simulink model "mvdc_path_matching"  (R2018b)
settings: configuration reference "Active" (kept outside this file)
undefined symbols (not defined in the file): P_VDC_ActivateHighPathDeviationDetection_b, P_VDC_CurvatureForesight_s, P_VDC_HeadingPathDeviationMax_rad, P_VDC_LateralPathDeviationMax_m, P_VDC_LocalFFCalculationActive_b, P_VDC_PathMatchForesight_m, P_VDC_PathMatchingTimeOut, P_VDC_PathMatchInterpPoints, P_VDC_PowertrainForesight_s, P_VDC_SmoothPathActive_b, P_VDC_SmoothPathWeights_DeltaCurvature, P_VDC_SmoothPathWeights_LatDeviation, tS, TUMPathMatchingState
libraries: simulink x5, rr_general x1
settings Model: DataDictionary=mvdc_path_matching.sldd  Creator=wischnewski  LastModifiedBy=ge34qer

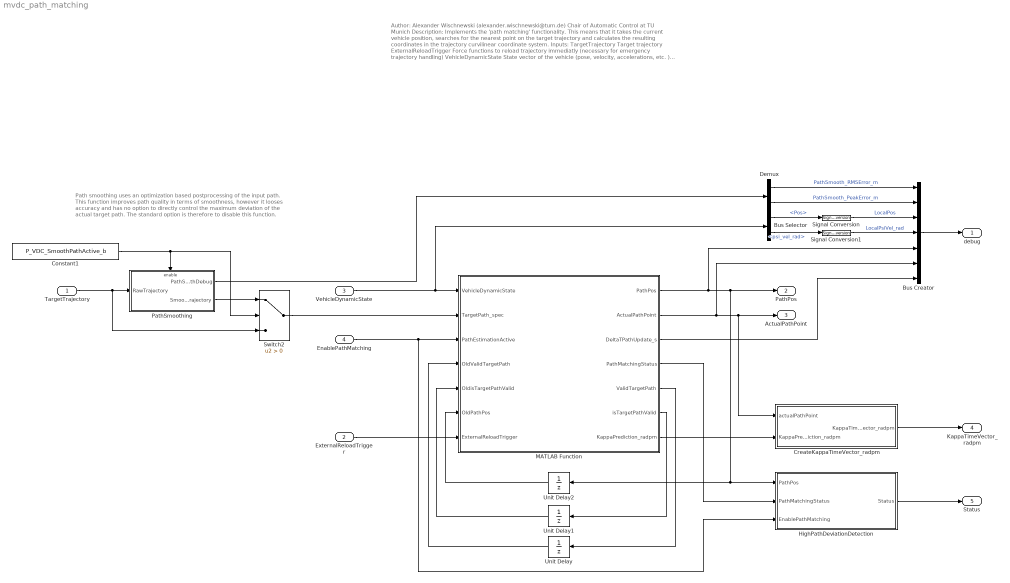
== system mvdc_path_matching ==
  note: Author: Alexander Wischnewski (alexander.wischnewski@tum.de)
      | Chair of Automatic Control at TU Munich
      |
      | Description: Implements the 'path matching' functionality. This means that it takes the current vehicle position, searches for
      | the nearest point on the target trajectory and calculates the resulting coordinates in the trajectory curvilinear
      | coordinate system.
      |
      | Inputs:
      | TargetTrajectory Target trajectory
      | ExternalReloadTrigger Force functions to reload trajectory immediatly (necessary for emergency trajectory handling)
      | VehicleDynamicState State vector of the vehicle (pose, velocity, accelerations, etc. )
      | EnablePathMatching Activates matching functionality
      |
      | Outputs:
      | debug debug bus
      | PathPos Vehicle position in path coordinates
      | ActualPathPoint Path on the target trajectory which is nearest to the vehicle
      | KappaTimeVector_radpm Vector which holds path curvature for a time window of +- 0.5sec
      | Status Function status used for state machine logic and diagnosis
  note: Path smoothing uses an optimization based postprocessing of the
      | input path. This function improves path quality in terms of smoothness,
      | however it looses accuracy and has no option to directly control the maximum deviation of the actual target path. The standard option is therefore to disable this function.
  TargetTrajectory : Inport  OutDataTypeStr=Bus: Trajectory  PortDimensions=1  Interpolate=off  BusOutputAsStruct=on
  ExternalReloadTrigger : Inport  Port=2  OutDataTypeStr=boolean  PortDimensions=1  BusOutputAsStruct=on
  VehicleDynamicState : Inport  Port=3  OutDataTypeStr=Bus: VehicleDynamicState  PortDimensions=1  BusOutputAsStruct=on
  EnablePathMatching : Inport  Port=4  OutDataTypeStr=boolean  PortDimensions=1  BusOutputAsStruct=on
  Bus Creator : BusCreator  Inputs=7  OutDataTypeStr=Bus: mvdc_path_matching_debug
  Bus Selector : BusSelector  OutputSignals=Pos,psi_vel_rad
  Constant1 : Constant  Value=P_VDC_SmoothPathActive_b
  CreateKappaTimeVector_radpm : Subsystem
  Demux : Demux  Outputs=2
  HighPathDeviationDetection : Subsystem
  MATLAB Function : MATLAB Function  TreatAsAtomicUnit=on
  PathSmoothing : Subsystem
  Signal Conversion : SignalConversion  OverrideOpt=off
  Signal Conversion1 : SignalConversion  OverrideOpt=off
  Switch2 : Switch  Criteria=u2 > Threshold
  Unit Delay : UnitDelay  SampleTime=-1
  Unit Delay1 : UnitDelay  SampleTime=-1
  Unit Delay2 : UnitDelay  SampleTime=-1
  debug : Outport  OutDataTypeStr=Bus: mvdc_path_matching_debug  PortDimensions=1  BusOutputAsStruct=on
  PathPos : Outport  Port=2  OutDataTypeStr=Bus: PathPos  PortDimensions=1  BusOutputAsStruct=on
  ActualPathPoint : Outport  Port=3  OutDataTypeStr=Bus: PathPoint  PortDimensions=1  BusOutputAsStruct=on
  KappaTimeVector_radpm : Outport  Port=4  PortDimensions=501
  Status : Outport  Port=5  OutDataTypeStr=Enum: TUMPathMatchingState  PortDimensions=1
  wires:
  MATLAB Function/1(PathPos) -> Unit Delay2/1, HighPathDeviationDetection/1(PathPos), PathPos/1, Bus Creator/5
  VehicleDynamicState/1 -> MATLAB Function/1(VehicleDynamicState), Bus Selector/1
  MATLAB Function/2(ActualPathPoint) -> CreateKappaTimeVector_radpm/1(actualPathPoint), ActualPathPoint/1, Bus Creator/6
  Bus Creator/1 -> debug/1
  MATLAB Function/3(DeltaTPathUpdate_s) -> Bus Creator/7
  HighPathDeviationDetection/1(Status) -> Status/1
  EnablePathMatching/1 -> HighPathDeviationDetection/3(EnablePathMatching), MATLAB Function/3(PathEstimationActive)
  Signal Conversion/1 -> Bus Creator/3  "LocalPos"
  MATLAB Function/5(ValidTargetPath) -> Unit Delay/1
  Unit Delay/1 -> MATLAB Function/4(OldValidTargetPath)
  MATLAB Function/6(isTargetPathValid) -> Unit Delay1/1
  Unit Delay1/1 -> MATLAB Function/5(OldisTargetPathValid)
  Unit Delay2/1 -> MATLAB Function/6(OldPathPos)
  Demux/1 -> Bus Creator/1  "PathSmooth_RMSError_m"
  Demux/2 -> Bus Creator/2  "PathSmooth_PeakError_m"
  Bus Selector/1 -> Signal Conversion/1  "<Pos>"
  Bus Selector/2 -> Signal Conversion1/1  "<psi_vel_rad>"
  Signal Conversion1/1 -> Bus Creator/4  "LocalPsiVel_rad"
  ExternalReloadTrigger/1 -> MATLAB Function/7(ExternalReloadTrigger)
  TargetTrajectory/1 -> Switch2/3, PathSmoothing/1(RawTrajectory)
  Constant1/1 -> Switch2/2, PathSmoothing/Enable
  PathSmoothing/2(SmoothTrajectory) -> Switch2/1
  Switch2/1 -> MATLAB Function/2(TargetPath_spec)
  PathSmoothing/1(PathSmoothDebug) -> Demux/1
  CreateKappaTimeVector_radpm/1(KappaTimeVector_radpm) -> KappaTimeVector_radpm/1
  MATLAB Function/7(KappaPrediction_radpm) -> CreateKappaTimeVector_radpm/2(KappaPrediction_radpm)
  MATLAB Function/4(PathMatchingStatus) -> HighPathDeviationDetection/2(PathMatchingStatus)

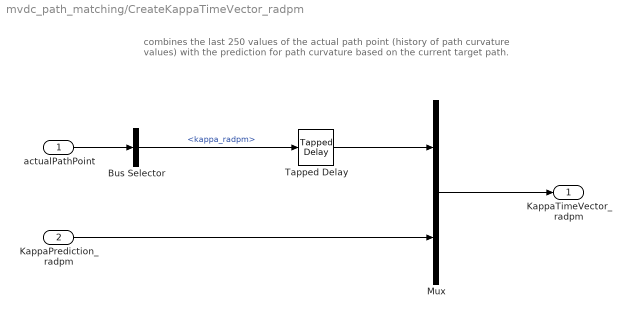
== system mvdc_path_matching/CreateKappaTimeVector_radpm ==
  note: combines the last 250 values of the actual path point (history of path curvature
      | values) with the prediction for path curvature based on the current target path.
  actualPathPoint : Inport
  KappaPrediction_radpm : Inport  Port=2
  Bus Selector : BusSelector  OutputSignals=kappa_radpm
  Mux : Mux  Inputs=2
  Tapped Delay : simulink/Discrete/Tapped Delay  vinit=0.0  samptime=-1  NumDelays=250  DelayOrder=Oldest  includeCurrent=off
  KappaTimeVector_radpm : Outport
  wires:
  Mux/1 -> KappaTimeVector_radpm/1
  KappaPrediction_radpm/1 -> Mux/2
  actualPathPoint/1 -> Bus Selector/1
  Bus Selector/1 -> Tapped Delay/1  "<kappa_radpm>"
  Tapped Delay/1 -> Mux/1

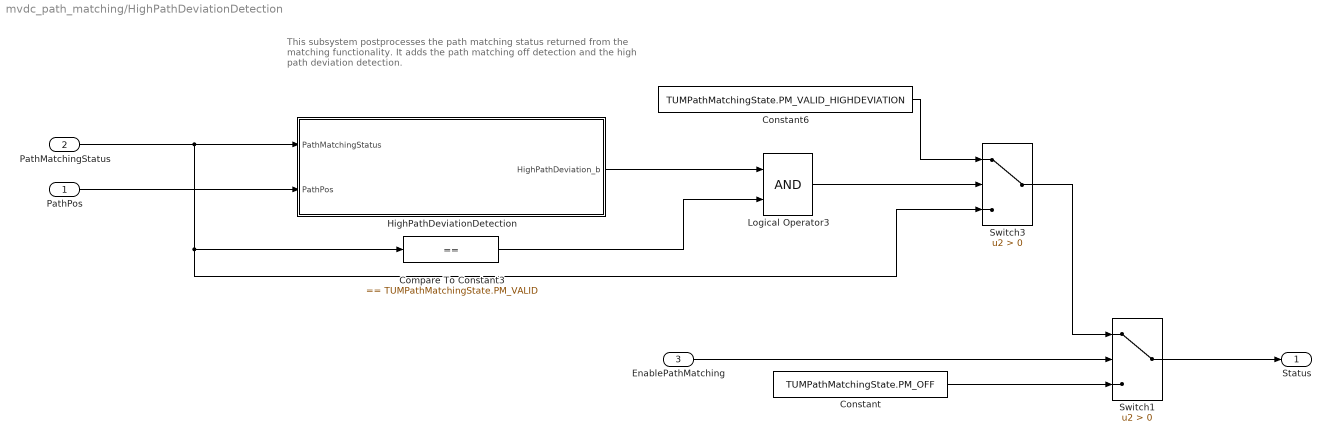
== system mvdc_path_matching/HighPathDeviationDetection ==
  note: This subsystem postprocesses the path matching status returned from the
      | matching functionality. It adds the path matching off detection and the
      | high path deviation detection.
  PathPos : Inport
  PathMatchingStatus : Inport  Port=2
  EnablePathMatching : Inport  Port=3
  Compare To Constant3 : simulink/Logic and Bit Operations/Compare To Constant  relop===  const=TUMPathMatchingState.PM_VALID  OutDataTypeStr=boolean
  Constant : Constant  Value=TUMPathMatchingState.PM_OFF
  Constant6 : Constant  Value=TUMPathMatchingState.PM_VALID_HIGHDEVIATION
  HighPathDeviationDetection : Subsystem
  Logical Operator3 : Logic  AllPortsSameDT=off  OutDataTypeStr=boolean
  Switch1 : Switch  Criteria=u2 > Threshold
  Switch3 : Switch  Criteria=u2 > Threshold
  Status : Outport  OutDataTypeStr=Enum: TUMPathMatchingState
  wires:
  EnablePathMatching/1 -> Switch1/2
  Constant/1 -> Switch1/3
  Switch1/1 -> Status/1
  Switch3/1 -> Switch1/1
  Logical Operator3/1 -> Switch3/2
  Compare To Constant3/1 -> Logical Operator3/2
  PathMatchingStatus/1 -> HighPathDeviationDetection/1(PathMatchingStatus), Switch3/3, Compare To Constant3/1
  PathPos/1 -> HighPathDeviationDetection/2(PathPos)
  HighPathDeviationDetection/1(HighPathDeviation_b) -> Logical Operator3/1
  Constant6/1 -> Switch3/1

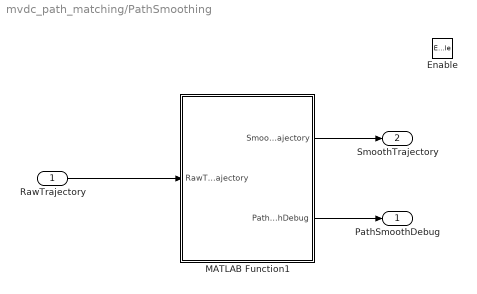
== system mvdc_path_matching/PathSmoothing ==
  RawTrajectory : Inport
  Enable : EnablePort
  MATLAB Function1 : MATLAB Function  TreatAsAtomicUnit=on
  PathSmoothDebug : Outport
  SmoothTrajectory : Outport  Port=2
  wires:
  MATLAB Function1/2(PathSmoothDebug) -> PathSmoothDebug/1
  MATLAB Function1/1(SmoothTrajectory) -> SmoothTrajectory/1
  RawTrajectory/1 -> MATLAB Function1/1(RawTrajectory)

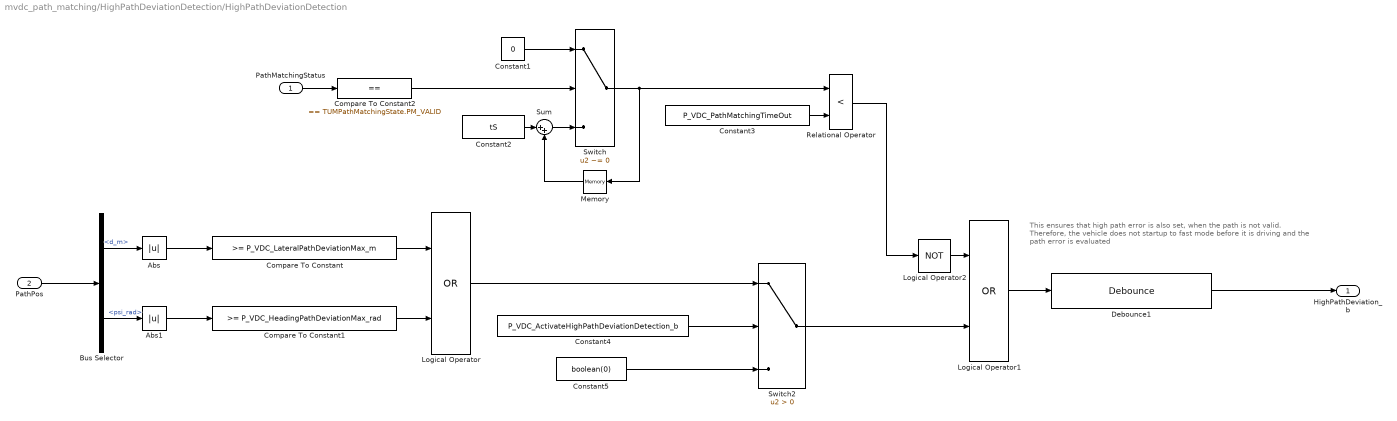
== system mvdc_path_matching/HighPathDeviationDetection/HighPathDeviationDetection ==
  note: This ensures that high path error is also set, when the path is not valid.
      | Therefore, the vehicle does not startup to fast mode before it is driving and
      | the path error is evaluated
  PathMatchingStatus : Inport
  PathPos : Inport  Port=2
  Abs : Abs
  Abs1 : Abs
  Bus Selector : BusSelector  OutputSignals=d_m,psi_rad
  Compare To Constant : simulink/Logic and Bit Operations/Compare To Constant  relop=>=  const=P_VDC_LateralPathDeviationMax_m  OutDataTypeStr=boolean
  Compare To Constant1 : simulink/Logic and Bit Operations/Compare To Constant  relop=>=  const=P_VDC_HeadingPathDeviationMax_rad  OutDataTypeStr=boolean
  Compare To Constant2 : simulink/Logic and Bit Operations/Compare To Constant  relop===  const=TUMPathMatchingState.PM_VALID  OutDataTypeStr=boolean
  Constant1 : Constant  Value=0
  Constant2 : Constant  Value=tS
  Constant3 : Constant  Value=P_VDC_PathMatchingTimeOut
  Constant4 : Constant  Value=P_VDC_ActivateHighPathDeviationDetection_b
  Constant5 : Constant  Value=boolean(0)
  Debounce1 : rr_general/Debounce  debounce_cycles=P_VDC_HighPathDeviationDebounce
  Logical Operator : Logic  Operator=OR  AllPortsSameDT=off  OutDataTypeStr=boolean
  Logical Operator1 : Logic  Operator=OR  AllPortsSameDT=off  OutDataTypeStr=boolean
  Logical Operator2 : Logic  Operator=NOT  AllPortsSameDT=off  OutDataTypeStr=boolean
  Memory : Memory  InitialCondition=P_VDC_PathMatchingTimeOut  InheritSampleTime=on
  Relational Operator : RelationalOperator  Operator=<  OutDataTypeStr=boolean  RndMeth=Nearest
  Sum : Sum  Inputs=|++
  Switch : Switch  Criteria=u2 ~= 0
  Switch2 : Switch  Criteria=u2 > Threshold
  HighPathDeviation_b : Outport
  wires:
  Switch/1 -> Memory/1, Relational Operator/1
  PathPos/1 -> Bus Selector/1
  Abs/1 -> Compare To Constant/1
  Logical Operator2/1 -> Logical Operator1/1
  Constant5/1 -> Switch2/3
  Logical Operator/1 -> Switch2/1
  Compare To Constant1/1 -> Logical Operator/2
  Constant4/1 -> Switch2/2
  Abs1/1 -> Compare To Constant1/1
  Compare To Constant/1 -> Logical Operator/1
  Sum/1 -> Switch/3
  Logical Operator1/1 -> Debounce1/1
  Relational Operator/1 -> Logical Operator2/1
  Bus Selector/1 -> Abs/1  "<d_m>"
  Switch2/1 -> Logical Operator1/2
  Debounce1/1 -> HighPathDeviation_b/1
  Bus Selector/2 -> Abs1/1  "<psi_rad>"
  Memory/1 -> Sum/2
  Constant3/1 -> Relational Operator/2
  Compare To Constant2/1 -> Switch/2
  Constant1/1 -> Switch/1
  Constant2/1 -> Sum/1
  PathMatchingStatus/1 -> Compare To Constant2/1

== matlab function mvdc_path_matching/PathSmoothing/MATLAB Function1 ==
  data: RawTrajectory input Bus: Trajectory; SmoothTrajectory output Bus: Trajectory; PathSmoothDebug output; P_VDC_SmoothPathWeights_LatDeviation parameter; P_VDC_SmoothPathWeights_DeltaCurvature parameter
function [SmoothTrajectory, PathSmoothDebug] = smoothRaceline(RawTrajectory, P_VDC_SmoothPathWeights_LatDeviation, P_VDC_SmoothPathWeights_DeltaCurvature)
  % wrapper function for smooth raceline
  [SmoothTrajectory, PathSmoothDebug] =...
  smoothRaceline(RawTrajectory, P_VDC_SmoothPathWeights_LatDeviation, P_VDC_SmoothPathWeights_DeltaCurvature);
end

== matlab function mvdc_path_matching/MATLAB Function ==
  data: VehicleDynamicState input Bus: VehicleDynamicState; TargetPath_spec input Bus: Trajectory; PathEstimationActive input boolean; OldValidTargetPath input Bus: Trajectory; OldisTargetPathValid input boolean; OldPathPos input Bus: PathPos; ExternalReloadTrigger input; PathPos output Bus: PathPos; tS parameter; ActualPathPoint output Bus: PathPoint; P_VDC_PathMatchInterpPoints parameter; P_VDC_PowertrainForesight_s parameter; P_VDC_CurvatureForesight_s parameter; P_VDC_LocalFFCalculationActive_b parameter; DeltaTPathUpdate_s output; P_VDC_PathMatchForesight_m parameter; PathMatchingStatus output Enum: TUMPathMatchingState; ValidTargetPath output Bus: Trajectory; isTargetPathValid output boolean size=1; KappaPrediction_radpm output size=251
function [PathPos, ActualPathPoint, DeltaTPathUpdate_s, PathMatchingStatus, ValidTargetPath, isTargetPathValid, KappaPrediction_radpm]  = mvdc_path_matching(VehicleDynamicState, TargetPath_spec, PathEstimationActive, OldValidTargetPath, OldisTargetPathValid, OldPathPos, ExternalReloadTrigger, tS, P_VDC_PathMatchInterpPoints, P_VDC_PowertrainForesight_s, P_VDC_CurvatureForesight_s, P_VDC_LocalFFCalculationActive_b, P_VDC_PathMatchForesight_m)
  [PathPos, ActualPathPoint, DeltaTPathUpdate_s, PathMatchingStatus, ValidTargetPath, isTargetPathValid, KappaPrediction_radpm] = local_path_matching(VehicleDynamicState, TargetPath_spec, PathEstimationActive, OldValidTargetPath, OldisTargetPathValid, OldPathPos, ExternalReloadTrigger, tS, P_VDC_PathMatchInterpPoints, P_VDC_PowertrainForesight_s, P_VDC_CurvatureForesight_s, P_VDC_LocalFFCalculationActive_b, P_VDC_PathMatchForesight_m);
end
